simulink model "OpenEndWinding"  (R2023b)
settings: Solver=VariableStepAuto  StartTime=0.0  StopTime=0.2  RelTol=1e-3  AbsTol=1e-3  EnableMultiTasking=on
values from neighbouring files (symbols this model uses):
  Amplitude = 0.9    [OpenEndWinding_sim.m]
  elec_freq = 5000/60* 4    (= 333.333333333)    [OpenEndWinding_sim.m]
  FSW = 36000    [OpenEndWinding_sim.m]
  Ki = C.Ki    [OpenEndWinding_sim.m]
  Kp = C.Kp    [OpenEndWinding_sim.m]
  Psi1_f = 0.05    [OpenEndWinding_sim.m]
  Rm = 10e-3    (= 0.01)    [OpenEndWinding_sim.m]
  sample_time = 1e-6    (= 1e-06)    [OpenEndWinding_sim.m]
libraries: nesl_utility x29, ee_lib x28, fl_lib x16, eeGeneralControl x5, spsRMSLib x5, spsTriangleGeneratorLib x2, simulink x2, eeLCFB1 x1, slpidlib x1, spspowerguiLib x1
(part 1 of 2)
settings Model: Creator=snow_  LastModifiedBy=snow_
settings SolverCC: AutoScaleAbsTol=off
settings DataIOCC: LimitDataPoints=on  MaxDataPoints=10000  ReturnWorkspaceOutputs=off
settings OptimizationCC: LifeSpan=inf
settings DebuggingCC: UnconnectedInputMsg=warning  UnconnectedOutputMsg=warning  UnconnectedLineMsg=warning  AllowSymbolicDim=off  SFUnexpectedBacktrackingDiag=warning  SFNoUnconditionalDefaultTransitionDiag=warning  SFExecutionAtInitializationDiag=none  ArithmeticOperatorsInVariantConditions=warning
settings ModelReferenceCC: EnableRefExpFcnMdlSchedulingChecks=on
settings SFSimCC: SimUseLocalCustomCode=off  CustomCodeUndefinedFunction=UseInterfaceOnly
settings RTWCC: RTWUseLocalCustomCode=off  DLArmComputeVersion=19.05
settings CodeAppCC: StateflowObjectComments=on
settings GRTTargetCC: TargetLangStandard=C89/C90 (ANSI)
settings ConfigComp: CovMetricSettings=dw  CovSaveCumulativeToWorkspaceVar=on  CovSaveSingleToWorkspaceVar=on  CovExternalEMLEnable=off  CovSFcnEnable=off
settings SimscapeCC: SimscapeLogType=all  SimscapeLogLimitData=off  SimscapeLogDataHistory=10000

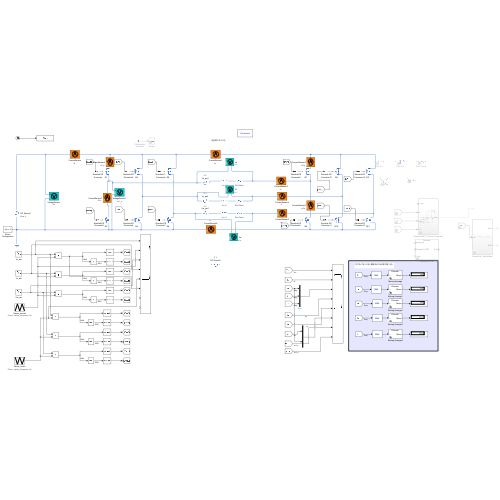
[thumbnail: Simulink's stored preview of the top-level diagram]
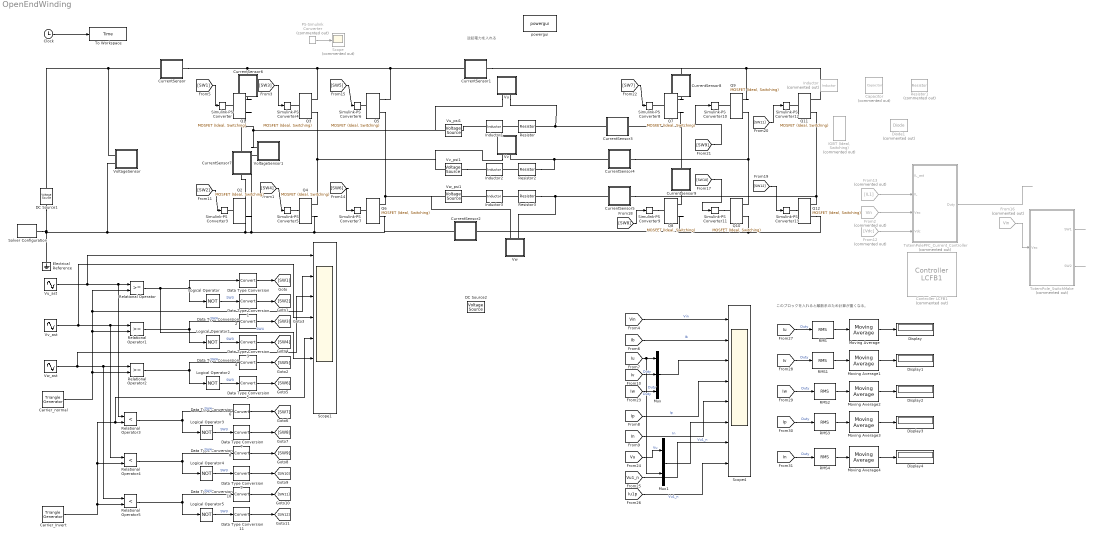
== system OpenEndWinding ==
  note: このブロックを入れると離散系のため計算が重くなる。
  note: 逆起電力を入れる
  Capacitor : ee_lib/Passive/Capacitor  Commented=on  cap_option=ee.enum.passive.capacitor.capOption.const  c=200e-6 F  Cvec=[1e-05, 1e-06] F  Vvec=[0, 10] V  CV_table_symmetry=1  f_vec=[1, 10] kHz  DFext_vec=[.8, 1.2]  enable_C_tol=0  averaging_period=0 s  C_tol=5  tol_distribution=1  nSigma=4  r=0 Ohm  g=0 1/Ohm  enable_operating_limits=0  operating_limit_action=2  max_working_voltage_range=[-25, 25] V  power_rating=1 W  enable_faults=ee.enum.enable.no  fault_action=simscape.enum.assert.action.none  Cscale_faulted=100  R_faulted=1e-3 Ohm  G_faulted=0 1/Ohm  tau_fault=1e-3 s  fault_trigger=ee.enum.faults.faultTrigger.temporal  t_fault=1 s  max_permissible_voltage_range=[-100, 100] V  t_fail_on_voltage=1 s  i_specify=off  i_priority=None  i=0 A  i_nominal_specify=off  i_nominal_unit=A  i_nominal_value=1  v_specify=off  v_priority=None  v=0 V  v_nominal_specify=off  v_nominal_unit=V  v_nominal_value=1  vc_specify=off  vc_priority=High  vc=0 V  vc_nominal_specify=off  vc_nominal_unit=V  vc_nominal_value=1
      settings: AttributesFormatString=%<c> H
  Carrier_Invert : spsTriangleGeneratorLib/Triangle Generator  Freq=carrier_frequency  Phase=180  Ts=sample_time
      settings: AttributesFormatString=Freq = %<Freq> Hz
  Carrier_normal : spsTriangleGeneratorLib/Triangle Generator  Freq=carrier_frequency  Phase=0  Ts=sample_time
      settings: AttributesFormatString=Freq = %<Freq> Hz
  Clock : Clock
  Controller LCFB1 : eeLCFB1/Controller LCFB1  Commented=on  pu_speed_reference=1  P_ref0=0.45  db=0  e_max=0.1  f_b=0  K_p=0  K_i=0.1  T_pelec=3.5  I_rmax=0.035  Ts=-1
      settings: LibrarySourceBlock=ee_sl_lib/Turbine-Governors/Controller LCFB1
  CurrentSensor : Subsystem  mask{Var=Ib, SampleTime=sample_time}
      mask prompts: Var "VariableName"; SampleTime "Simulink:blkprm_prompts:AllBlksSampleTime"
      settings: AttributesFormatString=%<Var>
      mask TypeOptions Var: Goto5/GotoTag | To Workspace1/VariableName
      mask TypeOptions SampleTime: To Workspace1/SampleTime
      mask DialogControl SampleTime Prompt: サンプル時間 (継承は -1):
      mask Display:
      | % disp("Current \n Sensor")
      | port_label('lconn', 1, '+')
      | port_label('rconn', 1, '-')
      | 
      | 
      | plot(-50,-35,50,50-15,...
      |     [0,9,18,24,29,30,29,24,18,9,0,-9,-18,-24,-29,-30,-29,-24,-18,-9,0],...
      |     0.8*[30,29,24,18,9,0,-9,-18,-24,-29,-30,-29,-24,-18,-9,0,9,18,24,29,30],...
      |     [-15,0,15],0.8*[-15,25,-15],...
      |     [-7,0,7],0.8*[5,5,5]);
  CurrentSensor1 : Subsystem  mask{Var=Ip, SampleTime=sample_time}
      mask prompts: Var "VariableName"; SampleTime "Simulink:blkprm_prompts:AllBlksSampleTime"
      settings: AttributesFormatString=%<Var>
      mask TypeOptions Var: Goto5/GotoTag | To Workspace1/VariableName
      mask TypeOptions SampleTime: To Workspace1/SampleTime
      mask DialogControl SampleTime Prompt: サンプル時間 (継承は -1):
      mask Display:
      | % disp("Current \n Sensor")
      | port_label('lconn', 1, '+')
      | port_label('rconn', 1, '-')
      | 
      | 
      | plot(-50,-35,50,50-15,...
      |     [0,9,18,24,29,30,29,24,18,9,0,-9,-18,-24,-29,-30,-29,-24,-18,-9,0],...
      |     0.8*[30,29,24,18,9,0,-9,-18,-24,-29,-30,-29,-24,-18,-9,0,9,18,24,29,30],...
      |     [-15,0,15],0.8*[-15,25,-15],...
      |     [-7,0,7],0.8*[5,5,5]);
  CurrentSensor2 : Subsystem  mask{Var=In, SampleTime=sample_time}
      mask prompts: Var "VariableName"; SampleTime "Simulink:blkprm_prompts:AllBlksSampleTime"
      settings: AttributesFormatString=%<Var>
      mask TypeOptions Var: Goto5/GotoTag | To Workspace1/VariableName
      mask TypeOptions SampleTime: To Workspace1/SampleTime
      mask DialogControl SampleTime Prompt: サンプル時間 (継承は -1):
      mask Display:
      | % disp("Current \n Sensor")
      | port_label('lconn', 1, '+')
      | port_label('rconn', 1, '-')
      | 
      | 
      | plot(-50,-35,50,50-15,...
      |     [0,9,18,24,29,30,29,24,18,9,0,-9,-18,-24,-29,-30,-29,-24,-18,-9,0],...
      |     0.8*[30,29,24,18,9,0,-9,-18,-24,-29,-30,-29,-24,-18,-9,0,9,18,24,29,30],...
      |     [-15,0,15],0.8*[-15,25,-15],...
      |     [-7,0,7],0.8*[5,5,5]);
  CurrentSensor3 : Subsystem  mask{Var=Iu, SampleTime=sample_time}
      mask prompts: Var "VariableName"; SampleTime "Simulink:blkprm_prompts:AllBlksSampleTime"
      settings: AttributesFormatString=%<Var>
      mask TypeOptions Var: Goto5/GotoTag | To Workspace1/VariableName
      mask TypeOptions SampleTime: To Workspace1/SampleTime
      mask DialogControl SampleTime Prompt: サンプル時間 (継承は -1):
      mask Display:
      | % disp("Current \n Sensor")
      | port_label('lconn', 1, '+')
      | port_label('rconn', 1, '-')
      | 
      | 
      | plot(-50,-35,50,50-15,...
      |     [0,9,18,24,29,30,29,24,18,9,0,-9,-18,-24,-29,-30,-29,-24,-18,-9,0],...
      |     0.8*[30,29,24,18,9,0,-9,-18,-24,-29,-30,-29,-24,-18,-9,0,9,18,24,29,30],...
      |     [-15,0,15],0.8*[-15,25,-15],...
      |     [-7,0,7],0.8*[5,5,5]);
  CurrentSensor4 : Subsystem  mask{Var=Iv, SampleTime=sample_time}
      mask prompts: Var "VariableName"; SampleTime "Simulink:blkprm_prompts:AllBlksSampleTime"
      settings: AttributesFormatString=%<Var>
      mask TypeOptions Var: Goto5/GotoTag | To Workspace1/VariableName
      mask TypeOptions SampleTime: To Workspace1/SampleTime
      mask DialogControl SampleTime Prompt: サンプル時間 (継承は -1):
      mask Display:
      | % disp("Current \n Sensor")
      | port_label('lconn', 1, '+')
      | port_label('rconn', 1, '-')
      | 
      | 
      | plot(-50,-35,50,50-15,...
      |     [0,9,18,24,29,30,29,24,18,9,0,-9,-18,-24,-29,-30,-29,-24,-18,-9,0],...
      |     0.8*[30,29,24,18,9,0,-9,-18,-24,-29,-30,-29,-24,-18,-9,0,9,18,24,29,30],...
      |     [-15,0,15],0.8*[-15,25,-15],...
      |     [-7,0,7],0.8*[5,5,5]);
  CurrentSensor5 : Subsystem  mask{Var=Iw, SampleTime=sample_time}
      mask prompts: Var "VariableName"; SampleTime "Simulink:blkprm_prompts:AllBlksSampleTime"
      settings: AttributesFormatString=%<Var>
      mask TypeOptions Var: Goto5/GotoTag | To Workspace1/VariableName
      mask TypeOptions SampleTime: To Workspace1/SampleTime
      mask DialogControl SampleTime Prompt: サンプル時間 (継承は -1):
      mask Display:
      | % disp("Current \n Sensor")
      | port_label('lconn', 1, '+')
      | port_label('rconn', 1, '-')
      | 
      | 
      | plot(-50,-35,50,50-15,...
      |     [0,9,18,24,29,30,29,24,18,9,0,-9,-18,-24,-29,-30,-29,-24,-18,-9,0],...
      |     0.8*[30,29,24,18,9,0,-9,-18,-24,-29,-30,-29,-24,-18,-9,0,9,18,24,29,30],...
      |     [-15,0,15],0.8*[-15,25,-15],...
      |     [-7,0,7],0.8*[5,5,5]);
  CurrentSensor6 : Subsystem  mask{Var=Iu1p, SampleTime=sample_time}
      mask prompts: Var "VariableName"; SampleTime "Simulink:blkprm_prompts:AllBlksSampleTime"
      settings: AttributesFormatString=%<Var>
      mask TypeOptions Var: Goto5/GotoTag | To Workspace1/VariableName
      mask TypeOptions SampleTime: To Workspace1/SampleTime
      mask DialogControl SampleTime Prompt: サンプル時間 (継承は -1):
      mask Display:
      | % disp("Current \n Sensor")
      | port_label('lconn', 1, '+')
      | port_label('rconn', 1, '-')
      | 
      | 
      | plot(-50,-35,50,50-15,...
      |     [0,9,18,24,29,30,29,24,18,9,0,-9,-18,-24,-29,-30,-29,-24,-18,-9,0],...
      |     0.8*[30,29,24,18,9,0,-9,-18,-24,-29,-30,-29,-24,-18,-9,0,9,18,24,29,30],...
      |     [-15,0,15],0.8*[-15,25,-15],...
      |     [-7,0,7],0.8*[5,5,5]);
  CurrentSensor7 : Subsystem  mask{Var=Iu1n, SampleTime=sample_time}
      mask prompts: Var "VariableName"; SampleTime "Simulink:blkprm_prompts:AllBlksSampleTime"
      settings: AttributesFormatString=%<Var>
      mask TypeOptions Var: Goto5/GotoTag | To Workspace1/VariableName
      mask TypeOptions SampleTime: To Workspace1/SampleTime
      mask DialogControl SampleTime Prompt: サンプル時間 (継承は -1):
      mask Display:
      | % disp("Current \n Sensor")
      | port_label('lconn', 1, '+')
      | port_label('rconn', 1, '-')
      | 
      | 
      | plot(-50,-35,50,50-15,...
      |     [0,9,18,24,29,30,29,24,18,9,0,-9,-18,-24,-29,-30,-29,-24,-18,-9,0],...
      |     0.8*[30,29,24,18,9,0,-9,-18,-24,-29,-30,-29,-24,-18,-9,0,9,18,24,29,30],...
      |     [-15,0,15],0.8*[-15,25,-15],...
      |     [-7,0,7],0.8*[5,5,5]);
  CurrentSensor8 : Subsystem  mask{Var=Iu2p, SampleTime=sample_time}
      mask prompts: Var "VariableName"; SampleTime "Simulink:blkprm_prompts:AllBlksSampleTime"
      settings: AttributesFormatString=%<Var>
      mask TypeOptions Var: Goto5/GotoTag | To Workspace1/VariableName
      mask TypeOptions SampleTime: To Workspace1/SampleTime
      mask DialogControl SampleTime Prompt: サンプル時間 (継承は -1):
      mask Display:
      | % disp("Current \n Sensor")
      | port_label('lconn', 1, '+')
      | port_label('rconn', 1, '-')
      | 
      | 
      | plot(-50,-35,50,50-15,...
      |     [0,9,18,24,29,30,29,24,18,9,0,-9,-18,-24,-29,-30,-29,-24,-18,-9,0],...
      |     0.8*[30,29,24,18,9,0,-9,-18,-24,-29,-30,-29,-24,-18,-9,0,9,18,24,29,30],...
      |     [-15,0,15],0.8*[-15,25,-15],...
      |     [-7,0,7],0.8*[5,5,5]);
  CurrentSensor9 : Subsystem  mask{Var=Iu2n, SampleTime=sample_time}
      mask prompts: Var "VariableName"; SampleTime "Simulink:blkprm_prompts:AllBlksSampleTime"
      settings: AttributesFormatString=%<Var>
      mask TypeOptions Var: Goto5/GotoTag | To Workspace1/VariableName
      mask TypeOptions SampleTime: To Workspace1/SampleTime
      mask DialogControl SampleTime Prompt: サンプル時間 (継承は -1):
      mask Display:
      | % disp("Current \n Sensor")
      | port_label('lconn', 1, '+')
      | port_label('rconn', 1, '-')
      | 
      | 
      | plot(-50,-35,50,50-15,...
      |     [0,9,18,24,29,30,29,24,18,9,0,-9,-18,-24,-29,-30,-29,-24,-18,-9,0],...
      |     0.8*[30,29,24,18,9,0,-9,-18,-24,-29,-30,-29,-24,-18,-9,0,9,18,24,29,30],...
      |     [-15,0,15],0.8*[-15,25,-15],...
      |     [-7,0,7],0.8*[5,5,5]);
  DC Source1 : ee_lib/Sources/Voltage Source  dc_voltage=Vbus V  ac_voltage=0 V  ac_shift=0 deg  ac_frequency=50 Hz  noise_mode=0  PSD=0 V^2/Hz  sample_time=1e-3 s  repeatability=1  user_seed=0  auto_seed=545404223  i_specify=off  i_priority=None  i=0 A  i_nominal_specify=off  i_nominal_unit=A  i_nominal_value=1  v_specify=off  v_priority=None  v=0 V  v_nominal_specify=off  v_nominal_unit=V  v_nominal_value=1
      settings: AttributesFormatString=%<dc_voltage> V
  DC Source2 : ee_lib/Sources/Voltage Source  dc_voltage=0 V  ac_voltage=Psi1_f * elec_freq*2*pi V  ac_shift=0 deg  ac_frequency=elec_freq Hz  noise_mode=0  PSD=0 V^2/Hz  sample_time=1e-3 s  repeatability=1  user_seed=0  auto_seed=4112460543  i_specify=off  i_priority=None  i=0 A  i_nominal_specify=off  i_nominal_unit=A  i_nominal_value=1  v_specify=off  v_priority=None  v=0 V  v_nominal_specify=off  v_nominal_unit=V  v_nominal_value=1
      settings: AttributesFormatString=%<dc_voltage> V
  Data Type Conversion{,1..11} (12 alike) : DataTypeConversion  SaturateOnIntegerOverflow=off  RndMeth=Floor
  Diode1 : ee_lib/Semiconductors & Converters/Diode  Commented=on  ModelType=ee.enum.diode.modelType.pwl  TableType=ee.enum.diode.tableType.IfMat  IfMat=[.07, .12, .19, 1.75, 4.24, 7.32, 11.2; .16, .3, .72, 2.14, 4.02, 6.35, 9.12] A  VfMat=[.9, 1.15, 1.25, 1.5, 1.75, 2.17, 2.6, 2.85; .58, .68, .75, 1.1, 1.38, 1.77, 2.27, 2.7] V  TjVec=[25, 125] degC  VfVec=[.5, .7, .9, 1.3, 1.7, 2.1, 2.5] V  IfVec=[.1, .2, .5, 1, 2, 4, 7, 10] A  Vf=0.6 V  Ron=0.3 Ohm  Goff=1e-8 S  prmExp=ee.enum.diode.expParam.useTwo  I12=[.0137, .545] A  V12=[.6, .7] V  RS=0 Ohm  Tmeas=25 degC  IS=1e-12 A  ec=1  I1=0.0137 A  V1=0.6 V  N_series=1  N_parallel=1  ZenerEnable=false  Rz=0.3 Ohm  BV=inf V  C_param=ee.enum.diode.capParam.fixed  CJ=5 pF  CJ0=5 pF  Vvec=[.1, 10, 100] V  Cvec=[3.5, 1, .4] pF  VJ=1 V  Mgrad=0.5  FC=0.5  Q_param=ee.enum.diode.recoveryParam.off  iRM=-7.15 A  iF=4 A  didt=-750 A/us  trr_factor=3  trr=115 ns  Qrr=150 s*nA  Vr=-600 V  Ls=150 nH  Erec=0.03 J  TT=50 ns  tau=100 ns  T_param=ee.enum.diode.temperatureParam.off  Tdevice=25 degC  I1_T2=0.245 A  V1_T2=0.5 V  IS_T2=1.25e-7 A  Tmeas2=125 degC  XTI_param=ee.enum.diode.xtiParam.pn  XTI=3  EG_param=ee.enum.diode.egapParam.material_si  EG=1.11 eV  dBVdT=0 V/K  enable_faults=ee.enum.enable.no  fault_action=simscape.enum.assert.action.none  fault_types=ee.enum.diode.faults.open  tau_fault=1e-3 s  IfMat_faulted=[.07, .12, .19, 1.75, 4.24, 7.32, 11.2; .16, .3, .72, 2.14, 4.02, 6.35, 9.12] A  VfMat_faulted=[.9, 1.15, 1.25, 1.5, 1.75, 2.17, 2.6, 2.85; .58, .68, .75, 1.1, 1.38, 1.77, 2.27, 2.7] V  VfVec_faulted=[.5, .7, .9, 1.3, 1.7, 2.1, 2.5] V  IfVec_faulted=[.1, .2, .5, 1, 2, 4, 7, 10] A  Ropen_faulted=1000 Ohm  Gshort_faulted=1000 1/Ohm  Vf_faulted=0.6 V  Ron_faulted=0.3 Ohm  Goff_faulted=1e-8 S  I12_faulted=[.0137, .545] A  V12_faulted=[.6, .7] V  IS_faulted=1e-12 A  ec_faulted=1  I1_faulted=0.0137 A  V1_faulted=0.6 V  RS_faulted=0 Ohm  Rz_faulted=0.3 Ohm  BV_faulted=inf V  Cscale_faulted=100  fault_trigger=ee.enum.faults.faultTrigger.temporal  t_fault=inf s  max_permissible_voltage=inf V  n_fail_on_voltage=1  max_permissible_current=inf A  t_fail_on_current=1 s  max_permissible_dVdt=inf V/s  enable_fault_input=simscape.enum.onoff.off  i_specify=off  i_priority=None  i=0 A  i_nominal_specify=off  i_nominal_unit=A  i_nominal_value=1  v_specify=off  v_priority=None  v=0 V  v_nominal_specify=off  v_nominal_unit=V  v_nominal_value=1  v_capacitor_specify=off  v_capacitor_priority=None  v_capacitor=0 V  v_capacitor_nominal_specify=off  v_capacitor_nominal_unit=V  v_capacitor_nominal_value=1  faulted_specify=off  faulted_priority=None  faulted=0  faulted_nominal_specify=off  faulted_nominal_unit=1  faulted_nominal_value=1  i_diode_specify=off  i_diode_priority=None  i_diode=0 A  i_diode_nominal_specify=off  i_diode_nominal_unit=A  i_diode_nominal_value=1  v_diode_specify=off  v_diode_priority=None  v_diode=0 V  v_diode_nominal_specify=off  v_diode_nominal_unit=V  v_diode_nominal_value=1  i_capacitor_specify=off  i_capacitor_priority=None  i_capacitor=0 A  i_capacitor_nominal_specify=off  i_capacitor_nominal_unit=A  i_capacitor_nominal_value=1  power_dissipated_specify=off  power_dissipated_priority=None  power_dissipated=0 W  power_dissipated_nominal_specify=off  power_dissipated_nominal_unit=W  power_dissipated_nominal_value=1  fidelity_level=ee.enum.diode.fidelity.includeChargeDyn  rec_loss_model=ee.enum.diode.reverseRecoveryModel.fixed  ErecVal=0 J  scaleWithIandV=false  ErecMat=zeros(2, 3) J  TjrecVec=[298.15, 398.15] K  IfrecVec=[.1, 1, 10] A  IrecVal=10 A  VrecVal=10 V  tFilter=1 / 1000 / 100 s  max_permissible_temperature=inf K  t_fail_on_temperature=1 s  thermal_network_parameterization=ee.enum.thermalNetworkTopology.junctionCase  Rth=[0, 10] K/W  Rth_Cauer=[1, 3, 10] K/W  Rth_Foster=[4, 6] K/W  thermal_mass_parameterization=ee.enum.thermalNetwork.timeconstant  thermal_mass=[0, 1] J/K  thermal_mass_Cauer=[.1, .3, 1] J/K  thermal_mass_Foster=[1.5, 3] J/K  thermal_time_constant=[0, 10] s  thermal_time_constant_Cauer=[1, 3, 10] s  thermal_time_constant_Foster=[6, 18] s  thermal_mass_initial_temperatures=[25, 25] degC  thermal_mass_initial_temperatures_Cauer=[25, 25, 25] degC  junction_thermal_mass=0.01 J/K  Tvec_initial_Foster=[25, 25, 25, 25] degC  no_thermal_network=0  junction_temperature_specify=off  junction_temperature_priority=None  junction_temperature=25 degC  junction_temperature_nominal_specify=off  junction_temperature_nominal_unit=degC  junction_temperature_nominal_value=1
      settings: InternalSimscapePortConfiguration="{\"Bottom\":[],\"Left\":[{\"id\":\"p\",\"label\":\"\",\"type\":\"foundation.electrical.electrical\"},{\"id\":\"H\",\"label\":\"\",\"type\":\"foundation.thermal.thermal\"}],\"Right\":[{\"id\":\"n\",\"label\":\"\",\"type\":\"foundation.electrical.electrical\"}],\"Top\":[]}"
  Display{,1..4} (5 alike) : Display
  Electrical Reference : fl_lib/Electrical/Electrical Elements/Electrical Reference
  From12 : From  Commented=on  GotoTag=Vdc  TagVisibility=global
  From13 : From  Commented=on  GotoTag=IL1  TagVisibility=global
  From16 : From  Commented=on  GotoTag=Vin  TagVisibility=global
  From2 : From  Commented=on  GotoTag=Vin  TagVisibility=global
  "IGBT (Ideal, Switching)" : ee_lib/Semiconductors & Converters/IGBT (Ideal, Switching)  Commented=on  port_option=ee.enum.controlport.elec  Vf=0.8 V  Ron=0.001 Ohm  Goff=1e-5 1/Ohm  Vth=6 V  diode_param=ee.enum.converters.protectiondiode.none  diode_Vf=0.8 V  diode_Ron=0.001 Ohm  diode_Goff=1e-5 1/Ohm  diode_C=50e-9 F  diode_iRM=-235 A  diode_iF=300 A  diode_idot=-50 A/us  diode_trr_param=ee.enum.converters.diodetrr.trr_factor  diode_trr_factor=3  diode_trr=15 us  diode_Qrr=1500 s*uA  ice_specify=off  ice_priority=None  ice=0 A  ice_nominal_specify=off  ice_nominal_unit=A  ice_nominal_value=1  vce_specify=off  vce_priority=None  vce=0 V  vce_nominal_specify=off  vce_nominal_unit=V  vce_nominal_value=1  vge_specify=off  vge_priority=None  vge=0 V  vge_nominal_specify=off  vge_nominal_unit=V  vge_nominal_value=1  thermal_loss_option=ee.enum.converters.thermalLossOption.constantvalues  Von_data=[0, .1, .6, .8, 1, 1.3, 1.6, 2, 2.4; 0, .1, .7, 1, 1.2, 1.5, 1.9, 2.4, 2.8] V  Tj=[298.15, 398.15] K  Iout_data=[0, .1, 1, 5, 10, 20, 40, 70, 100] A  Eon_data=[0, .0024, .024, .12, .2, .48, 1.04, 2.16, 3.24; 0, .003, .03, .15, .25, .6, 1.3, 2.7, 4.05] * 1e-3 J  Eoff_data=[0, .0007, .0066, .033, .066, .17, .33, .83, 1.5; 0, .001, .01, .05, .1, .25, .5, 1.2, 2.2] * 1e-3 J  Eon_data_3D=[zeros(2, 9, 3)] J  Eoff_data_3D=[zeros(2, 9, 3)] J  Tj_loss=[298.15, 398.15] K  Iout_data_loss=[0, .1, 1, 5, 10, 20, 40, 70, 100] A  tabulateWithVce=false  Vce_loss=[0, 150, 300] V  Eon_scalar=22.86e-3 J  Eoff_scalar=17.14e-3 J  Voff=300 V  Iout_scalar=600 A  useCurrentFromPreviousCycle=true  useVoltageFromPreviousCycle=true  diodeModelType=ee.enum.converters.diodeModelType.pwl  diodeTableType=ee.enum.diode.tableType.IfMat  diode_IfMat=[.07, .12, .19, 1.75, 4.24, 7.32, 11.2; .16, .3, .72, 2.14, 4.02, 6.35, 9.12] A  diode_VfMat=[.9, 1.15, 1.25, 1.5, 1.75, 2.17, 2.6, 2.85; .58, .68, .75, 1.1, 1.38, 1.77, 2.27, 2.7] V  diode_TjVec=[25, 125] degC  diode_VfVec=[.5, .7, .9, 1.3, 1.7, 2.1, 2.5] V  diode_IfVec=[.1, .2, .5, 1, 2, 4, 7, 10] A  diode_Vr=-600 V  diode_Ls=150 nH  diode_Erec=0.03 J  diode_rec_loss_model=ee.enum.diode.reverseRecoveryModel.fixed  diode_ErecVal=0 J  diode_scaleWithIandV=false  diode_ErecMat=zeros(2, 3) J  diode_TjrecVec=[298.15, 398.15] K  diode_IfrecVec=[.1, 1, 10] A  diode_IrecVal=10 A  diode_VrecVal=10 V  diode_tFilter=1 / 1000 / 100 s  thermal_network_parameterization=ee.enum.thermalNetworkTopology.external  Rth=[.08, .5] K/W  Rth_Cauer=[.08, .1, .5] K/W  Rth_Foster=[.08, .14, .22, .16] K/W  thermal_mass_parameterization=ee.enum.thermalNetwork.timeconstant  thermal_mass=[.01, .5] J/K  thermal_mass_Cauer=[.01, .1, .5] J/K  thermal_mass_Foster=[.001, .005, .05, .5] J/K  thermal_time_constant=[.001, .2] s  thermal_time_constant_Cauer=[.001, .1, .2] s  thermal_time_constant_Foster=[7e-05, .0007, .01, .08] s  thermal_mass_initial_temperatures=[25, 25] degC  thermal_mass_initial_temperatures_Cauer=[25, 25, 25] degC  junction_thermal_mass=0.01 J/K  Tvec_initial_Foster=[25, 25, 25, 25] degC  no_thermal_network=0  junction_temperature_specify=off  junction_temperature_priority=None  junction_temperature=25 degC  junction_temperature_nominal_specify=off  junction_temperature_nominal_unit=degC  junction_temperature_nominal_value=1  Qj_specify=off  Qj_priority=None  Qj=0 W  Qj_nominal_specify=off  Qj_nominal_unit=W  Qj_nominal_value=1  accumulatedSwitchingLosses_specify=off  accumulatedSwitchingLosses_priority=None  accumulatedSwitchingLosses=0 J
      settings: InternalSimscapePortConfiguration="{\"Bottom\":[],\"Left\":[{\"id\":\"G_elec\",\"label\":\"\",\"type\":\"foundation.electrical.electrical\"},{\"id\":\"H\",\"label\":\"\",\"type\":\"foundation.thermal.thermal\"}],\"Right\":[{\"id\":\"C\",\"label\":\"\",\"type\":\"foundation.electrical.electrical\"},{\"id\":\"E\",\"label\":\"\",\"type\":\"foundation.electrical.electrical\"}],\"Top\":[]}"
  Inductor : ee_lib/Passive/Inductor  Commented=on  l=200e-6 H  enable_L_tol=0  L_tol=20  tol_distribution=1  nSigma=4  r=0 Ohm  g=1e-9 1/Ohm  enable_operating_limits=0  operating_limit_action=2  max_working_current=1 A  power_rating=1 W  enable_faults=ee.enum.enable.no  fault_action=simscape.enum.assert.action.none  lambdaPercent=50  k_faulted=0.9999  turnsShort=0  openCct=0  groundShort=0  groundShortG=0 1/Ohm  tau_fault=1e-3 s  fault_trigger=ee.enum.faults.faultTrigger.temporal  t_fault=1 s  max_permissible_voltage=100 V  n_fail_on_voltage=1  max_permissible_current=1 A  t_fail_on_current=1 s  i_L_specify=off  i_L_priority=High  i_L=0 A  i_L_nominal_specify=off  i_L_nominal_unit=A  i_L_nominal_value=1
      settings: AttributesFormatString=%<l> H
  Inductor1 : ee_lib/Passive/Inductor  l=Lm H  enable_L_tol=0  L_tol=20  tol_distribution=1  nSigma=4  r=0 Ohm  g=1e-9 1/Ohm  enable_operating_limits=0  operating_limit_action=2  max_working_current=1 A  power_rating=1 W  enable_faults=ee.enum.enable.no  fault_action=simscape.enum.assert.action.none  lambdaPercent=50  k_faulted=0.9999  turnsShort=0  openCct=0  groundShort=0  groundShortG=0 1/Ohm  tau_fault=1e-3 s  fault_trigger=ee.enum.faults.faultTrigger.temporal  t_fault=1 s  max_permissible_voltage=100 V  n_fail_on_voltage=1  max_permissible_current=1 A  t_fail_on_current=1 s  i_L_specify=off  i_L_priority=High  i_L=0 A  i_L_nominal_specify=off  i_L_nominal_unit=A  i_L_nominal_value=1
      settings: AttributesFormatString=%<l> H
  Inductor2 : ee_lib/Passive/Inductor  l=Lm H  enable_L_tol=0  L_tol=20  tol_distribution=1  nSigma=4  r=0 Ohm  g=1e-9 1/Ohm  enable_operating_limits=0  operating_limit_action=2  max_working_current=1 A  power_rating=1 W  enable_faults=ee.enum.enable.no  fault_action=simscape.enum.assert.action.none  lambdaPercent=50  k_faulted=0.9999  turnsShort=0  openCct=0  groundShort=0  groundShortG=0 1/Ohm  tau_fault=1e-3 s  fault_trigger=ee.enum.faults.faultTrigger.temporal  t_fault=1 s  max_permissible_voltage=100 V  n_fail_on_voltage=1  max_permissible_current=1 A  t_fail_on_current=1 s  i_L_specify=off  i_L_priority=High  i_L=0 A  i_L_nominal_specify=off  i_L_nominal_unit=A  i_L_nominal_value=1
      settings: AttributesFormatString=%<l> H
  Inductor3 : ee_lib/Passive/Inductor  l=Lm H  enable_L_tol=0  L_tol=20  tol_distribution=1  nSigma=4  r=0 Ohm  g=1e-9 1/Ohm  enable_operating_limits=0  operating_limit_action=2  max_working_current=1 A  power_rating=1 W  enable_faults=ee.enum.enable.no  fault_action=simscape.enum.assert.action.none  lambdaPercent=50  k_faulted=0.9999  turnsShort=0  openCct=0  groundShort=0  groundShortG=0 1/Ohm  tau_fault=1e-3 s  fault_trigger=ee.enum.faults.faultTrigger.temporal  t_fault=1 s  max_permissible_voltage=100 V  n_fail_on_voltage=1  max_permissible_current=1 A  t_fail_on_current=1 s  i_L_specify=off  i_L_priority=High  i_L=0 A  i_L_nominal_specify=off  i_L_nominal_unit=A  i_L_nominal_value=1
      settings: AttributesFormatString=%<l> H
  Logical Operator{,1..5} (6 alike) : Logic  Operator=NOT  AllPortsSameDT=off  OutDataTypeStr=boolean
  Moving Average{,1..4} (5 alike) : eeGeneralControl/Moving Average  VariantControl=Variant1  LabelModeActiveChoice=Discrete  f=elec_freq  x0=0  BufferSize=8192  Ts=sample_time
      settings: LibrarySourceBlock=ee_sl_lib/General Control/Moving Average
  Mux : Mux  Inputs=3
  Mux1 : Mux  Inputs=2
  PS-Simulink Converter : nesl_utility/PS-Simulink Converter  Commented=on  PhysicalDomain=network_engine_domain  SubClassName=ps_output  LeftPortType=input  RightPortType=output  PseudoPeriodic=off  Frequencies=[]  VectorFormat=1-D array  Unit=inherit  AffineConversion=off
  Q{1..12} (12 alike) : ee_lib/Semiconductors & Converters/MOSFET (Ideal, Switching)  port_option=ee.enum.controlport.ps  Rds=Ron Ohm  Goff=1e-6 1/Ohm  Vth=0.5 V  diode_param=ee.enum.converters.protectiondiode.nodynamics  diode_Vf=Vf V  diode_Ron=Rdiode Ohm  diode_Goff=1e-5 1/Ohm  diode_C=50e-9 F  diode_iRM=-235 A  diode_iF=300 A  diode_idot=-50 A/us  diode_trr_param=ee.enum.converters.diodetrr.trr_factor  diode_trr_factor=3  diode_trr=15 us  diode_Qrr=1500 s*uA  ids_specify=off  ids_priority=None  ids=0 A  ids_nominal_specify=off  ids_nominal_unit=A  ids_nominal_value=1  vds_specify=off  vds_priority=None  vds=0 V  vds_nominal_specify=off  vds_nominal_unit=V  vds_nominal_value=1  vgs_specify=off  vgs_priority=None  vgs=0 V  vgs_nominal_specify=off  vgs_nominal_unit=V  vgs_nominal_value=1  thermal_loss_option=ee.enum.converters.thermalLossOption.constantvalues  Von_data=[0, 1.8, 3.2, 6, 10, 16; 0, 2, 5.5, 9.5, 15, 25] V  Tj=[298.15, 448.15] K  Iout_data=[0, 20, 40, 60, 80, 100] A  Eon_data=[0, 55.04, 124.57, 235.53, 362.12; 0, 71.25, 161.25, 304.88, 468.75] * 1e-6 J  Eoff_data=[0, 18, 30, 56.1, 76.5; 0, 22.5, 37.5, 70.13, 95.63] * 1e-6 J  Eon_data_3D=[zeros(2, 5, 3)] J  Eoff_data_3D=[zeros(2, 5, 3)] J  Tj_loss=[298.15, 448.15] K  Iout_data_loss=[0, 10, 20, 30, 40] A  tabulateWithVds=false  Vds_loss=[0, 150, 300] V  Eon_scalar=22.86e-3 J  Eoff_scalar=17.14e-3 J  Voff=300 V  Iout_scalar=600 A  useCurrentFromPreviousCycle=false  useVoltageFromPreviousCycle=false  diodeModelType=ee.enum.converters.diodeModelType.pwl  diodeTableType=ee.enum.diode.tableType.IfMat  diode_IfMat=[.07, .12, .19, 1.75, 4.24, 7.32, 11.2; .16, .3, .72, 2.14, 4.02, 6.35, 9.12] A  diode_VfMat=[.9, 1.15, 1.25, 1.5, 1.75, 2.17, 2.6, 2.85; .58, .68, .75, 1.1, 1.38, 1.77, 2.27, 2.7] V  diode_TjVec=[25, 125] degC  diode_VfVec=[.5, .7, .9, 1.3, 1.7, 2.1, 2.5] V  diode_IfVec=[.1, .2, .5, 1, 2, 4, 7, 10] A  diode_Vr=-600 V  diode_Ls=150 nH  diode_Erec=0.03 J  diode_rec_loss_model=ee.enum.diode.reverseRecoveryModel.fixed  diode_ErecVal=0 J  diode_scaleWithIandV=true  diode_ErecMat=zeros(2, 3) J  diode_TjrecVec=[298.15, 398.15] K  diode_IfrecVec=[.1, 1, 10] A  diode_IrecVal=10 A  diode_VrecVal=10 V  diode_tFilter=1 / 1000 / 100 s  thermal_network_parameterization=ee.enum.thermalNetworkTopology.external  Rth=[.03, .2] K/W  Rth_Cauer=[.03, .1, .2] K/W  Rth_Foster=[.03, .2] K/W  thermal_mass_parameterization=ee.enum.thermalNetwork.timeconstant  thermal_mass=[3, 25] J/K  thermal_mass_Cauer=[3, 10, 25] J/K  thermal_mass_Foster=[33, 50] J/K  thermal_time_constant=[.1, 5] s  thermal_time_constant_Cauer=[.1, 1, 5] s  thermal_time_constant_Foster=[1, 10] s  thermal_mass_initial_temperatures=[25, 25] degC  thermal_mass_initial_temperatures_Cauer=[25, 25, 25] degC  junction_thermal_mass=0.1 J/K  Tvec_initial_Foster=[25, 25, 25, 25] degC  no_thermal_network=0  junction_temperature_specify=off  junction_temperature_priority=None  junction_temperature=25 degC  junction_temperature_nominal_specify=off  junction_temperature_nominal_unit=degC  junction_temperature_nominal_value=1  Qj_specify=off  Qj_priority=None  Qj=0 W  Qj_nominal_specify=off  Qj_nominal_unit=W  Qj_nominal_value=1  accumulatedSwitchingLosses_specify=off  accumulatedSwitchingLosses_priority=None  accumulatedSwitchingLosses=0 J
  RMS{,1..4} (5 alike) : spsRMSLib/RMS  TrueRMS=on  Freq=elec_freq  RMSInit=0  Ts=sample_time
  Relational Operator : RelationalOperator  OutDataTypeStr=boolean  RndMeth=Simplest  InputSameDT=off
  Relational Operator1 : RelationalOperator  OutDataTypeStr=boolean  RndMeth=Simplest  InputSameDT=off
  Relational Operator2 : RelationalOperator  OutDataTypeStr=boolean  RndMeth=Simplest  InputSameDT=off
  Relational Operator3 : RelationalOperator  Operator=<  OutDataTypeStr=boolean  RndMeth=Simplest  InputSameDT=off
  Relational Operator4 : RelationalOperator  Operator=<  OutDataTypeStr=boolean  RndMeth=Simplest  InputSameDT=off
  Relational Operator5 : RelationalOperator  Operator=<  OutDataTypeStr=boolean  RndMeth=Simplest  InputSameDT=off
  Resistor : ee_lib/Passive/Resistor  R=Rm Ohm  enable_R_tol=0  R_tol=5  tol_distribution=1  nSigma=4  enable_operating_limits=0  operating_limit_action=2  power_rating=1 W  max_working_voltage=100 V  enable_faults=ee.enum.enable.no  fault_action=simscape.enum.assert.action.none  R_faulted=inf Ohm  fault_trigger=ee.enum.faults.faultTrigger.temporal  t_fault=1 s  max_permissible_current=1 A  t_fail_on_current=1 s  noise_mode=0  Tdevice=25 degC  sample_time=1e-3 s  repeatability=1  user_seed=0  auto_seed=3890346746  faulted_specify=off  faulted_priority=None  faulted=0  power_derating_T1=70 degC  power_derating_T2=155 degC  operating_temperature_range_vec=[-50, 150] degC  alpha=3.93e-3 1/K  Tmeas=25 degC  thermal_mass=100 J/K  temperature_specify=off  temperature_priority=High  temperature=298.15 K  temperature_nominal_specify=off  temperature_nominal_unit=K  temperature_nominal_value=1
      settings: AttributesFormatString=%<R> Ohms
  Resistor1 : ee_lib/Passive/Resistor  Commented=on  R=20e-3 Ohm  enable_R_tol=0  R_tol=5  tol_distribution=1  nSigma=4  enable_operating_limits=0  operating_limit_action=2  power_rating=1 W  max_working_voltage=100 V  enable_faults=ee.enum.enable.no  fault_action=simscape.enum.assert.action.none  R_faulted=inf Ohm  fault_trigger=ee.enum.faults.faultTrigger.temporal  t_fault=1 s  max_permissible_current=1 A  t_fail_on_current=1 s  noise_mode=0  Tdevice=25 degC  sample_time=1e-3 s  repeatability=1  user_seed=0  auto_seed=1403765601  faulted_specify=off  faulted_priority=None  faulted=0  power_derating_T1=70 degC  power_derating_T2=155 degC  operating_temperature_range_vec=[-50, 150] degC  alpha=3.93e-3 1/K  Tmeas=25 degC  thermal_mass=100 J/K  temperature_specify=off  temperature_priority=High  temperature=298.15 K  temperature_nominal_specify=off  temperature_nominal_unit=K  temperature_nominal_value=1
      settings: AttributesFormatString=%<R> Ohms
  Resistor2 : ee_lib/Passive/Resistor  R=Rm Ohm  enable_R_tol=0  R_tol=5  tol_distribution=1  nSigma=4  enable_operating_limits=0  operating_limit_action=2  power_rating=1 W  max_working_voltage=100 V  enable_faults=ee.enum.enable.no  fault_action=simscape.enum.assert.action.none  R_faulted=inf Ohm  fault_trigger=ee.enum.faults.faultTrigger.temporal  t_fault=1 s  max_permissible_current=1 A  t_fail_on_current=1 s  noise_mode=0  Tdevice=25 degC  sample_time=1e-3 s  repeatability=1  user_seed=0  auto_seed=1196140742  faulted_specify=off  faulted_priority=None  faulted=0  power_derating_T1=70 degC  power_derating_T2=155 degC  operating_temperature_range_vec=[-50, 150] degC  alpha=3.93e-3 1/K  Tmeas=25 degC  thermal_mass=100 J/K  temperature_specify=off  temperature_priority=High  temperature=298.15 K  temperature_nominal_specify=off  temperature_nominal_unit=K  temperature_nominal_value=1
      settings: AttributesFormatString=%<R> Ohms
  Resistor3 : ee_lib/Passive/Resistor  R=Rm Ohm  enable_R_tol=0  R_tol=5  tol_distribution=1  nSigma=4  enable_operating_limits=0  operating_limit_action=2  power_rating=1 W  max_working_voltage=100 V  enable_faults=ee.enum.enable.no  fault_action=simscape.enum.assert.action.none  R_faulted=inf Ohm  fault_trigger=ee.enum.faults.faultTrigger.temporal  t_fault=1 s  max_permissible_current=1 A  t_fail_on_current=1 s  noise_mode=0  Tdevice=25 degC  sample_time=1e-3 s  repeatability=1  user_seed=0  auto_seed=2348838240  faulted_specify=off  faulted_priority=None  faulted=0  power_derating_T1=70 degC  power_derating_T2=155 degC  operating_temperature_range_vec=[-50, 150] degC  alpha=3.93e-3 1/K  Tmeas=25 degC  thermal_mass=100 J/K  temperature_specify=off  temperature_priority=High  temperature=298.15 K  temperature_nominal_specify=off  temperature_nominal_unit=K  temperature_nominal_value=1
      settings: AttributesFormatString=%<R> Ohms
  Scope : Scope  Commented=on
  Scope1 : Scope  NumInputPorts=8
  Scope4 : Scope  NumInputPorts=8
  Simulink-PS Converter{,3..13} (12 alike) : nesl_utility/Simulink-PS Converter  PhysicalDomain=network_engine_domain  SubClassName=ps_input  LeftPortType=input  RightPortType=output  PseudoPeriodic=off  Frequencies=[]  NoiseDistribution=none  NoiseParameters=[]  Unit=V  AffineConversion=off  FilteringAndDerivatives=provide  SimscapeFilterOrder=1  InputFilterTimeConstant=0.001  UdotUserProvided=0
  Solver Configuration : nesl_utility/Solver Configuration  PhysicalDomain=network_engine_domain  SubClassName=solver  LeftPortType=input  RightPortType=generic  Tones=[]  Harmonics=[]  SimulateNoise=off  Profile=off  UseLocalSampling=off  EnableSwitchedLinearOptims=on  FrequencyDomain=off  UseCCode=off  RelTol=0.001  AbsTol=1e-06  MinStep=1e-09  ToWorkspace=off  RevertToSquareIcSolve=off  NumHomotopyIterations=100  PhasorMode=off  PhasorModeNumHarmonics=1  ConsistencySolver=NEWTON_FTOL  IndexReductionMethod=DerivativeReplacement  DoDC=off  ResidualTolerance=1e-09  ConsistencyTolSource=GLOBAL  ConsistencyAbsTol=0.001  ConsistencyRelTol=0.001  ConsistencyTolFactor=0.001  UseLocalSolver=off  LocalSolverChoice=NE_BACKWARD_EULER_ADVANCER  ResolveIndetEquations=on  FunctionEvalNumThread=1  LocalSolverSampleTime=0.001  DoFixedCost=off  MaxNonlinIter=3  MaxModeIter=2  ComputeImpulses=off  ImpulseIterations=2  LinearAlgebra=auto  LinearAlgebraNumThread=0  EquationFormulation=NE_TIME_EF  DelaysMemoryBudget=1024  AutomaticFiltering=on  FilteringTimeConstant=0.001  PartitionStorageMethod=AS_NEEDED  PartitionMemoryBudget=1024  PartitionMethod=ROBUST  MultibodyUseLocalSolver=off  MultibodyLocalSolverChoice=ODE1  MultibodyLocalSolverSampleTime=0.001
  To Workspace : ToWorkspace  VariableName=Time  SampleTime=sample_time
  TotemPolePFC_Current_Controller : Subsystem  Commented=on
  TotemPole_SwitchMake : Subsystem  Commented=on
  VoltageSensor : Subsystem  mask{VariableName=Vin, SampleTime=sample_time}
      mask prompts: VariableName "Simulink:blkprm_prompts:ToWksVarName"; SampleTime "Simulink:blkprm_prompts:AllBlksSampleTime"
      settings: AttributesFormatString=%<VariableName>
      mask TypeOptions VariableName: To Workspace1/VariableName | Goto5/GotoTag
      mask TypeOptions SampleTime: To Workspace1/SampleTime
      mask DialogControl VariableName Prompt: 変数名:
      mask DialogControl SampleTime Prompt: サンプル時間 (継承は -1):
      mask Display:
      | %disp("Voltage \n Sensor")
      | port_label('lconn', 1, '+')
      | port_label('lconn', 2, '-')
      | 
      | plot(-50,-35,50,50-15,...
      |     [0,9,18,24,29,30,29,24,18,9,0,-9,-18,-24,-29,-30,-29,-24,-18,-9,0],...
      |     0.8*[30,29,24,18,9,0,-9,-18,-24,-29,-30,-29,-24,-18,-9,0,9,18,24,29,30],...
      |     [-15,0,15],0.8*[15,-20,15]);
  VoltageSensor1 : Subsystem  mask{VariableName=Vu1_n, SampleTime=sample_time}
      mask prompts: VariableName "Simulink:blkprm_prompts:ToWksVarName"; SampleTime "Simulink:blkprm_prompts:AllBlksSampleTime"
      settings: AttributesFormatString=%<VariableName>
      mask TypeOptions VariableName: To Workspace1/VariableName | Goto5/GotoTag
      mask TypeOptions SampleTime: To Workspace1/SampleTime
      mask DialogControl VariableName Prompt: 変数名:
      mask DialogControl SampleTime Prompt: サンプル時間 (継承は -1):
      mask Display:
      | %disp("Voltage \n Sensor")
      | port_label('lconn', 1, '+')
      | port_label('lconn', 2, '-')
      | 
      | plot(-50,-35,50,50-15,...
      |     [0,9,18,24,29,30,29,24,18,9,0,-9,-18,-24,-29,-30,-29,-24,-18,-9,0],...
      |     0.8*[30,29,24,18,9,0,-9,-18,-24,-29,-30,-29,-24,-18,-9,0,9,18,24,29,30],...
      |     [-15,0,15],0.8*[15,-20,15]);
  Vu : Subsystem  mask{VariableName=Vu, SampleTime=sample_time}
      mask prompts: VariableName "Simulink:blkprm_prompts:ToWksVarName"; SampleTime "Simulink:blkprm_prompts:AllBlksSampleTime"
      settings: AttributesFormatString=%<VariableName>
      mask TypeOptions VariableName: To Workspace1/VariableName | Goto5/GotoTag
      mask TypeOptions SampleTime: To Workspace1/SampleTime
      mask DialogControl VariableName Prompt: 変数名:
      mask DialogControl SampleTime Prompt: サンプル時間 (継承は -1):
      mask Display:
      | %disp("Voltage \n Sensor")
      | port_label('lconn', 1, '+')
      | port_label('lconn', 2, '-')
      | 
      | plot(-50,-35,50,50-15,...
      |     [0,9,18,24,29,30,29,24,18,9,0,-9,-18,-24,-29,-30,-29,-24,-18,-9,0],...
      |     0.8*[30,29,24,18,9,0,-9,-18,-24,-29,-30,-29,-24,-18,-9,0,9,18,24,29,30],...
      |     [-15,0,15],0.8*[15,-20,15]);
  "Vu_ast " : Sin  Amplitude=Amplitude  Frequency=2*pi*elec_freq  SampleTime=0
  Vu_psi1 : ee_lib/Sources/Voltage Source  dc_voltage=0 V  ac_voltage=Psi1_f*elec_freq*2*pi V  ac_shift=0 deg  ac_frequency=elec_freq Hz  noise_mode=0  PSD=0 V^2/Hz  sample_time=1e-3 s  repeatability=1  user_seed=0  auto_seed=676943032  i_specify=off  i_priority=None  i=0 A  i_nominal_specify=off  i_nominal_unit=A  i_nominal_value=1  v_specify=off  v_priority=None  v=0 V  v_nominal_specify=off  v_nominal_unit=V  v_nominal_value=1
      settings: AttributesFormatString=%<dc_voltage> V
  Vv : Subsystem  mask{VariableName=Vv, SampleTime=sample_time}
      mask prompts: VariableName "Simulink:blkprm_prompts:ToWksVarName"; SampleTime "Simulink:blkprm_prompts:AllBlksSampleTime"
      settings: AttributesFormatString=%<VariableName>
      mask TypeOptions VariableName: To Workspace1/VariableName | Goto5/GotoTag
      mask TypeOptions SampleTime: To Workspace1/SampleTime
      mask DialogControl VariableName Prompt: 変数名:
      mask DialogControl SampleTime Prompt: サンプル時間 (継承は -1):
      mask Display:
      | %disp("Voltage \n Sensor")
      | port_label('lconn', 1, '+')
      | port_label('lconn', 2, '-')
      | 
      | plot(-50,-35,50,50-15,...
      |     [0,9,18,24,29,30,29,24,18,9,0,-9,-18,-24,-29,-30,-29,-24,-18,-9,0],...
      |     0.8*[30,29,24,18,9,0,-9,-18,-24,-29,-30,-29,-24,-18,-9,0,9,18,24,29,30],...
      |     [-15,0,15],0.8*[15,-20,15]);
  Vv_ast : Sin  Amplitude=Amplitude  Frequency=2*pi*elec_freq  Phase=pi*2/3  SampleTime=0
  Vv_psi1 : ee_lib/Sources/Voltage Source  dc_voltage=0 V  ac_voltage=Psi1_f*elec_freq*2*pi V  ac_shift=120 deg  ac_frequency=elec_freq Hz  noise_mode=0  PSD=0 V^2/Hz  sample_time=1e-3 s  repeatability=1  user_seed=0  auto_seed=2084672538  i_specify=off  i_priority=None  i=0 A  i_nominal_specify=off  i_nominal_unit=A  i_nominal_value=1  v_specify=off  v_priority=None  v=0 V  v_nominal_specify=off  v_nominal_unit=V  v_nominal_value=1
      settings: AttributesFormatString=%<dc_voltage> V
  Vw : Subsystem  mask{VariableName=Vw, SampleTime=sample_time}
      mask prompts: VariableName "Simulink:blkprm_prompts:ToWksVarName"; SampleTime "Simulink:blkprm_prompts:AllBlksSampleTime"
      settings: AttributesFormatString=%<VariableName>
      mask TypeOptions VariableName: To Workspace1/VariableName | Goto5/GotoTag
      mask TypeOptions SampleTime: To Workspace1/SampleTime
      mask DialogControl VariableName Prompt: 変数名:
      mask DialogControl SampleTime Prompt: サンプル時間 (継承は -1):
      mask Display:
      | %disp("Voltage \n Sensor")
      | port_label('lconn', 1, '+')
      | port_label('lconn', 2, '-')
      | 
      | plot(-50,-35,50,50-15,...
      |     [0,9,18,24,29,30,29,24,18,9,0,-9,-18,-24,-29,-30,-29,-24,-18,-9,0],...
      |     0.8*[30,29,24,18,9,0,-9,-18,-24,-29,-30,-29,-24,-18,-9,0,9,18,24,29,30],...
      |     [-15,0,15],0.8*[15,-20,15]);
  Vw_ast : Sin  Amplitude=Amplitude  Frequency=2*pi*elec_freq  Phase=pi*4/3  SampleTime=0
  Vw_psi1 : ee_lib/Sources/Voltage Source  dc_voltage=0 V  ac_voltage=Psi1_f*elec_freq*2*pi V  ac_shift=240 deg  ac_frequency=elec_freq Hz  noise_mode=0  PSD=0 V^2/Hz  sample_time=1e-3 s  repeatability=1  user_seed=0  auto_seed=3437178441  i_specify=off  i_priority=None  i=0 A  i_nominal_specify=off  i_nominal_unit=A  i_nominal_value=1  v_specify=off  v_priority=None  v=0 V  v_nominal_specify=off  v_nominal_unit=V  v_nominal_value=1
      settings: AttributesFormatString=%<dc_voltage> V
  powergui : spspowerguiLib/powergui  Priority=1  SimulationMode=Continuous  SampleTime=50e-6  frequency=60  Iterations=50  frequencyindice=50  Pbase=100e6  ErrMax=1e-4  UnitsV=kV  UnitsW=MW  buscounter=0  FunctionMessages=off  echomessages=off  EnableUseOfTLC=off  CurrentSourceSwitches=off  DisableSnubberDevices=off  DisableRonSwitches=off  DisableVfSwitches=off  DisplayEquations=off  AutomaticDiscreteSolvers=off  SolverType=Tustin/Backward Euler (TBE)  Interpol=off  ExternalGateDelay=off  methode=off  Ts=100  x0status=blocks  SPID=on  SwTol=0  HookPort=off  NonlinearTolerance=1e-4  nMaxIteration=100  ContinueOnMaxIteration=off  RestoreLinks=warning  ResistiveCurrentMeasurement=off  Frange=[0:2:500]  Ylog=off  Xlog=on  ShowGrid=off  save=off  variable=ZData  structure=0  ZoomFFT=off  StartTime=0.0  cycles=1  DisplayStyle=1  fundamental=60  FreqAxis=off  MaxFrequency=1000  frequencyindicesteady=1  RmsSteady=1  display=off
  wires:
  PS-Simulink Converter/1 -> Scope/1
  [SW1] -> Simulink-PS Converter/1
  From13/1 -> TotemPolePFC_Current_Controller/2(IL)
  From2/1 -> TotemPolePFC_Current_Controller/3(Vac)
  From12/1 -> TotemPolePFC_Current_Controller/4(Vdc)
  TotemPolePFC_Current_Controller/1(Duty) -> ?
  From16/1 -> TotemPole_SwitchMake/1(Vac)
  TotemPole_SwitchMake/2(SW2) -> ?
  TotemPole_SwitchMake/1(SW1) -> ?
  Clock/1 -> To Workspace/1
  [SW2] -> Simulink-PS Converter3/1
  [SW4] -> Simulink-PS Converter5/1
  [SW3] -> Simulink-PS Converter4/1
  [SW5] -> Simulink-PS Converter6/1
  [SW6] -> Simulink-PS Converter7/1
  [SW11] -> Simulink-PS Converter12/1
  [SW12] -> Simulink-PS Converter13/1
  [SW9] -> Simulink-PS Converter10/1
  [SW10] -> Simulink-PS Converter11/1
  [SW8] -> Simulink-PS Converter9/1
  [SW7] -> Simulink-PS Converter8/1
  [Vin] -> Scope4/1  "Vin"
  [Ip] -> Scope4/4  "Ip"
  [In] -> Scope4/5  "In"
  [Ib] -> Scope4/2  "Ib"
  [Iu] -> Mux1/2, Mux/1  "Duty"
  [Iv] -> Mux/2  "Duty"
  [Iw] -> Mux/3  "Duty"
  Mux/1 -> Scope4/3
  [Vu] -> Mux1/1  "Vu"
  Logical Operator/1 -> Data Type Conversion1/1  "SW3"
  Data Type Conversion1/1 -> [SW2]
  Data Type Conversion/1 -> [SW1]
  "Vu_ast "/1 -> Scope1/1, Relational Operator3/1, Relational Operator/1
  Relational Operator/1 -> Scope1/6, Data Type Conversion/1, Logical Operator/1  "SW4"
  Logical Operator1/1 -> Data Type Conversion3/1  "SW3"
  Data Type Conversion2/1 -> [SW3]
  Vv_ast/1 -> Scope1/4, Relational Operator4/1, Relational Operator1/1
  Relational Operator1/1 -> Data Type Conversion2/1, Logical Operator1/1  "SW4"
  Data Type Conversion3/1 -> [SW4]
  Data Type Conversion5/1 -> [SW6]
  Logical Operator2/1 -> Data Type Conversion5/1  "SW3"
  Relational Operator2/1 -> Data Type Conversion4/1, Logical Operator2/1  "SW4"
  Data Type Conversion4/1 -> [SW5]
  Carrier_normal/1 -> Relational Operator2/2, Relational Operator/2, Scope1/2, Relational Operator1/2
  Vw_ast/1 -> Scope1/3, Relational Operator5/1, Relational Operator2/1
  Data Type Conversion9/1 -> [SW10]
  Logical Operator4/1 -> Data Type Conversion9/1  "SW3"
  Relational Operator4/1 -> Data Type Conversion8/1, Logical Operator4/1  "SW4"
  Data Type Conversion8/1 -> [SW9]
  Logical Operator3/1 -> Data Type Conversion7/1  "SW3"
  Data Type Conversion10/1 -> [SW11]
  Logical Operator5/1 -> Data Type Conversion11/1  "SW3"
  Data Type Conversion11/1 -> [SW12]
  Relational Operator5/1 -> Data Type Conversion10/1, Logical Operator5/1  "SW4"
  Data Type Conversion6/1 -> [SW7]
  Relational Operator3/1 -> Data Type Conversion6/1, Logical Operator3/1  "SW4"
  Data Type Conversion7/1 -> [SW8]
  Carrier_Invert/1 -> Relational Operator5/2, Relational Operator4/2, Scope1/5, Relational Operator3/2
  [Vu1_n] -> Scope4/7  "Vu1_n"
  [Iu1p] -> Scope4/8  "Vu1_n"
  Mux1/1 -> Scope4/6
  [Iu] -> RMS/1  "Duty"
  [Iv] -> RMS1/1  "Duty"
  [Iw] -> RMS2/1  "Duty"
  Moving Average/1 -> Display/1
  Moving Average1/1 -> Display1/1
  Moving Average2/1 -> Display2/1
  RMS/1 -> Moving Average/1
  RMS1/1 -> Moving Average1/1
  RMS2/1 -> Moving Average2/1
  [Ip] -> RMS3/1  "Duty"
  RMS3/1 -> Moving Average3/1
  Moving Average3/1 -> Display3/1
  [In] -> RMS4/1  "Duty"
  Moving Average4/1 -> Display4/1
  RMS4/1 -> Moving Average4/1
  connections:
  VoltageSensor/LConn2 -- VoltageSensor1/LConn2 -- CurrentSensor2/RConn1 -- Q6/RConn2 -- Q4/RConn2 -- Q2/RConn2 -- DC Source1/RConn1 -- Solver Configuration/RConn1 -- Electrical Reference/LConn1
  VoltageSensor/LConn1 -- DC Source1/LConn1 -- CurrentSensor/LConn1
  CurrentSensor1/RConn1 -- CurrentSensor8/LConn1 -- Q9/RConn1 -- Q11/RConn1
  Q1/LConn1 -- Simulink-PS Converter/RConn1
  Resistor/LConn1 -- Inductor1/RConn1
  Simulink-PS Converter3/RConn1 -- Q2/LConn1
  Vv_psi1/RConn1 -- Inductor2/LConn1
  Q3/LConn1 -- Simulink-PS Converter4/RConn1
  Simulink-PS Converter5/RConn1 -- Q4/LConn1
  Simulink-PS Converter7/RConn1 -- Q6/LConn1
  Q5/LConn1 -- Simulink-PS Converter6/RConn1
  CurrentSensor9/RConn1 -- Q8/RConn1
  Q11/LConn1 -- Simulink-PS Converter12/RConn1
  Q9/LConn1 -- Simulink-PS Converter10/RConn1
  Simulink-PS Converter13/RConn1 -- Q12/LConn1
  Simulink-PS Converter11/RConn1 -- Q10/LConn1
  Simulink-PS Converter9/RConn1 -- Q8/LConn1
  Q7/LConn1 -- Simulink-PS Converter8/RConn1
  CurrentSensor7/RConn1 -- Q2/RConn1
  Q5/RConn2 -- Vw/LConn1 -- Vw_psi1/LConn1 -- Q6/RConn1
  Q9/RConn2 -- CurrentSensor4/RConn1 -- Q10/RConn1
  Q11/RConn2 -- CurrentSensor5/RConn1 -- Q12/RConn1
  Resistor2/LConn1 -- Inductor2/RConn1
  Resistor3/LConn1 -- Inductor3/RConn1
  CurrentSensor/RConn1 -- CurrentSensor6/LConn1 -- Q3/RConn1 -- Q5/RConn1 -- CurrentSensor1/LConn1
  Q10/RConn2 -- Q8/RConn2 -- CurrentSensor2/LConn1 -- Q12/RConn2
  CurrentSensor3/LConn1 -- Vu/LConn2 -- Resistor/RConn1
  Resistor2/RConn1 -- CurrentSensor4/LConn1 -- Vv/LConn2
  Resistor3/RConn1 -- CurrentSensor5/LConn1 -- Vw/LConn2
  Q1/RConn1 -- CurrentSensor6/RConn1
  VoltageSensor1/LConn1 -- Vu/LConn1 -- Vu_psi1/LConn1 -- Q1/RConn2 -- CurrentSensor7/LConn1
  Q7/RConn1 -- CurrentSensor8/RConn1
  Q7/RConn2 -- CurrentSensor9/LConn1 -- CurrentSensor3/RConn1
  Q3/RConn2 -- Vv/LConn1 -- Vv_psi1/LConn1 -- Q4/RConn1
  Inductor1/LConn1 -- Vu_psi1/RConn1
  Inductor3/LConn1 -- Vw_psi1/RConn1

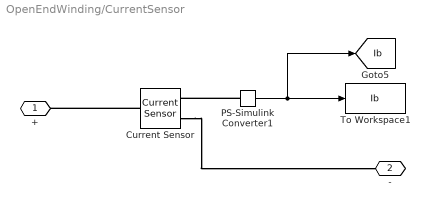
== system OpenEndWinding/CurrentSensor ==
  Current Sensor : fl_lib/Electrical/Electrical Sensors/Current Sensor
  PS-Simulink Converter1 : nesl_utility/PS-Simulink Converter  PhysicalDomain=network_engine_domain  SubClassName=ps_output  LeftPortType=input  RightPortType=output  PseudoPeriodic=off  Frequencies=[]  VectorFormat=1-D array  Unit=A  AffineConversion=off
  To Workspace1 : ToWorkspace  VariableName=Ib  SampleTime=SampleTime
  + : PMIOPort  Side=Left
  - : PMIOPort  Port=2  Side=Right
  tag scope: Ib=global
  wires:
  PS-Simulink Converter1/1 -> [Ib], To Workspace1/1
  connections:
  Current Sensor/RConn2 -- -/RConn1
  Current Sensor/LConn1 -- +/RConn1
  PS-Simulink Converter1/LConn1 -- Current Sensor/RConn1

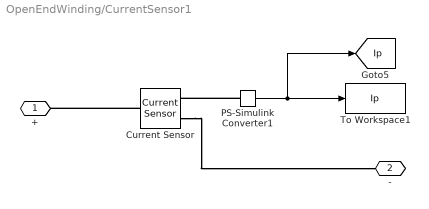
== system OpenEndWinding/CurrentSensor1 ==
  Current Sensor : fl_lib/Electrical/Electrical Sensors/Current Sensor
  PS-Simulink Converter1 : nesl_utility/PS-Simulink Converter  PhysicalDomain=network_engine_domain  SubClassName=ps_output  LeftPortType=input  RightPortType=output  PseudoPeriodic=off  Frequencies=[]  VectorFormat=1-D array  Unit=A  AffineConversion=off
  To Workspace1 : ToWorkspace  VariableName=Ip  SampleTime=SampleTime
  + : PMIOPort  Side=Left
  - : PMIOPort  Port=2  Side=Right
  tag scope: Ip=global
  wires:
  PS-Simulink Converter1/1 -> [Ip], To Workspace1/1
  connections:
  Current Sensor/RConn2 -- -/RConn1
  Current Sensor/LConn1 -- +/RConn1
  PS-Simulink Converter1/LConn1 -- Current Sensor/RConn1
